simulink model "WDGBrakeTimeCalc"  (R2024a)
settings: configuration reference "csMultiInstance" (kept outside this file)
undefined symbols (not defined in the file or in its folder): driver_decel, FB_decel, PB1_decel, PB2_decel, StopTime_Max, StopTime_Min, timeMargin, timeToReact, Ts, Velocity_Max
Description:
  | Software unit for Stopping time calculation
settings Model: DataDictionary=DD_WDGBrakeTimeCalc.sldd  EnableAccessToBaseWorkspace=off  Creator=The MathWorks, Inc.  LastModifiedBy=The MathWorks, Inc.
settings ConfigSetRef: SourceName=csMultiInstance

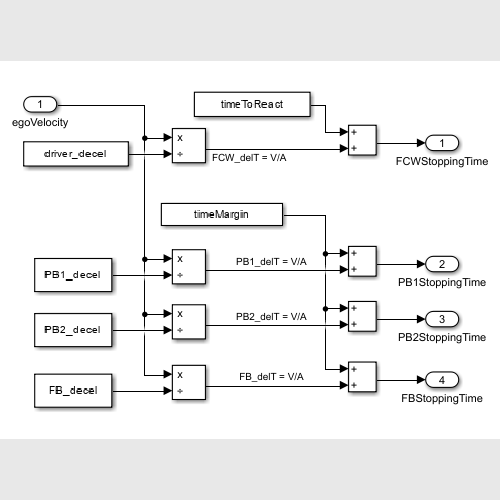
[thumbnail: Simulink's stored preview of the top-level diagram]
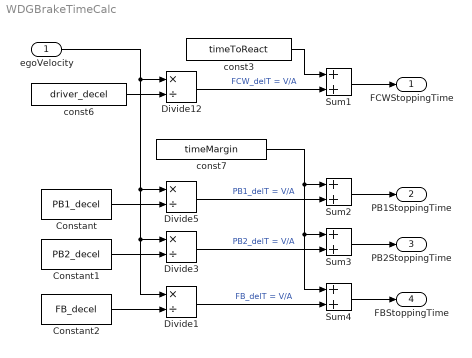
== system WDGBrakeTimeCalc ==
  egoVelocity : Inport  OutMin=0  OutMax=Velocity_Max  OutDataTypeStr=Velocity_DType  Unit=m/s  PortDimensions=Velocity_Dimensions  SampleTime=Ts
  Constant : Constant  Value=PB1_decel
  Constant1 : Constant  Value=PB2_decel
  Constant2 : Constant  Value=FB_decel
  Divide{1,3,5,12} (4 alike) : Product  Inputs=*/
  Sum{1..4} (4 alike) : Sum
  const3 : Constant  Value=timeToReact  SampleTime=-1
  const6 : Constant  Value=driver_decel  SampleTime=-1
  const7 : Constant  Value=timeMargin  SampleTime=-1
  FCWStoppingTime : Outport  OutMin=StopTime_Min  OutMax=StopTime_Max  OutDataTypeStr=StopTime_DType  Unit=s  PortDimensions=StopTime_Dimensions  SampleTime=Ts  VectorParamsAs1DForOutWhenUnconnected=off
  PB1StoppingTime : Outport  Port=2  OutMin=StopTime_Min  OutMax=StopTime_Max  OutDataTypeStr=StopTime_DType  Unit=s  PortDimensions=StopTime_Dimensions  SampleTime=Ts  VectorParamsAs1DForOutWhenUnconnected=off
  PB2StoppingTime : Outport  Port=3  OutMin=StopTime_Min  OutMax=StopTime_Max  OutDataTypeStr=StopTime_DType  Unit=s  PortDimensions=StopTime_Dimensions  SampleTime=Ts  VectorParamsAs1DForOutWhenUnconnected=off
  FBStoppingTime : Outport  Port=4  OutMin=StopTime_Min  OutMax=StopTime_Max  OutDataTypeStr=StopTime_DType  Unit=s  PortDimensions=StopTime_Dimensions  SampleTime=Ts  VectorParamsAs1DForOutWhenUnconnected=off
  wires:
  Sum3/1 -> PB2StoppingTime/1
  Constant2/1 -> Divide1/2
  const6/1 -> Divide12/2
  Constant1/1 -> Divide3/2
  const7/1 -> Sum3/1, Sum4/1, Sum2/1
  Constant/1 -> Divide5/2
  Sum2/1 -> PB1StoppingTime/1
  egoVelocity/1 -> Divide12/1, Divide5/1, Divide3/1, Divide1/1
  Divide5/1 -> Sum2/2  "PB1_delT = V/A"
  Sum4/1 -> FBStoppingTime/1
  Divide1/1 -> Sum4/2  "FB_delT = V/A"
  Divide12/1 -> Sum1/2  "FCW_delT = V/A"
  Sum1/1 -> FCWStoppingTime/1
  const3/1 -> Sum1/1
  Divide3/1 -> Sum3/2  "PB2_delT = V/A"
